simulink model "Bai04"  (R2018a)
settings: Solver=VariableStepAuto  StartTime=0.0  StopTime=5  RelTol=1e-3
settings Model: Creator=Ngoc Cute  LastModifiedBy=Ngoc Cute

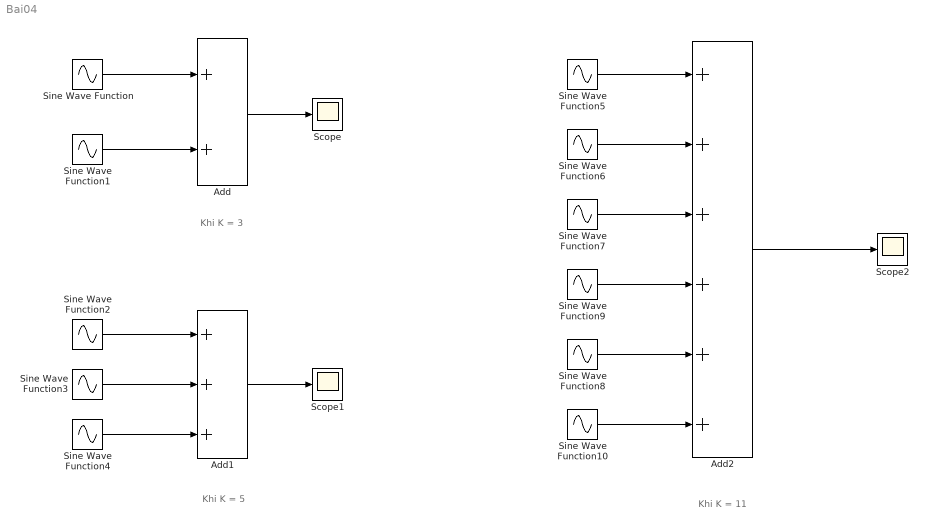
== system Bai04 ==
  note: Khi K = 3
  note: Khi K = 5
  note: Khi K = 11
  Add : Sum
  Add1 : Sum  Inputs=+++
  Add2 : Sum  Inputs=++++++
  Scope : Scope
  Scope1 : Scope
  Scope2 : Scope
  Sine Wave Function : Sin  Frequency=2*pi  SampleTime=0.000001
  Sine Wave Function1 : Sin  Amplitude=1/3  Frequency=2*pi*3  SampleTime=0.000001
  Sine Wave Function10 : Sin  Amplitude=1/11  Frequency=2*pi*11  SampleTime=0.000001
  Sine Wave Function2 : Sin  Frequency=2*pi  SampleTime=0.000001
  Sine Wave Function3 : Sin  Amplitude=1/3  Frequency=2*pi*3  SampleTime=0.000001
  Sine Wave Function4 : Sin  Amplitude=1/5  Frequency=2*pi*5  SampleTime=0.000001
  Sine Wave Function5 : Sin  Frequency=2*pi  SampleTime=0.000001
  Sine Wave Function6 : Sin  Amplitude=1/3  Frequency=2*pi*3  SampleTime=0.000001
  Sine Wave Function7 : Sin  Amplitude=1/5  Frequency=2*pi*5  SampleTime=0.000001
  Sine Wave Function8 : Sin  Amplitude=1/9  Frequency=2*pi*9  SampleTime=0.000001
  Sine Wave Function9 : Sin  Amplitude=1/7  Frequency=2*pi*7  SampleTime=0.000001
  wires:
  Sine Wave Function/1 -> Add/1
  Sine Wave Function1/1 -> Add/2
  Add/1 -> Scope/1
  Sine Wave Function3/1 -> Add1/2
  Add1/1 -> Scope1/1
  Sine Wave Function2/1 -> Add1/1
  Sine Wave Function4/1 -> Add1/3
  Sine Wave Function6/1 -> Add2/2
  Sine Wave Function5/1 -> Add2/1
  Add2/1 -> Scope2/1
  Sine Wave Function7/1 -> Add2/3
  Sine Wave Function9/1 -> Add2/4
  Sine Wave Function8/1 -> Add2/5
  Sine Wave Function10/1 -> Add2/6
